simulink model "controlevento"  (Simulink 7.5)
settings: Solver=ode45  StartTime=0.0  StopTime=10000  RelTol=1e-3
values from neighbouring files (symbols this model uses):
  DL = tan(gamma0)*cos(sigma0)    [estressemain.m]    (also in main1.m)
  g = 9.81    [estressemain.m]    (also in main1.m)
  h0 = 5000    [estressemain.m]    (also in main1.m)
  href = 800    [estressemain.m]    (also in main1.m = 1000)
  meanw1 = 7    [estressemain.m]    (also in main1.m)
  meanw2 = 6    [estressemain.m]    (also in main1.m)
  meanw3 = 5    [estressemain.m]    (also in main1.m)
  meanw4 = 4    [estressemain.m]    (also in main1.m)
  meanw5 = 3    [estressemain.m]    (also in main1.m)
  psi0 = 360*(pi/180)    (= 6.28318530718)    [estressemain.m]    (also in main1.m)
  raioref = 400    [estressemain.m]    (also in main1.m)
  rhoH = 1.112    [estressemain.m]    (also in main1.m)
  rhoHo = 1.225    [estressemain.m]    (also in main1.m)
  Vo = 9    [estressemain.m]    (also in main1.m)
  wn = 1    [estressemain.m]    (also in main1.m = 150)
  x0 = 1000+i*rand    [estressemain.m]    (also in main1.m = 1000)
  xf = 0    [estressemain.m]    (also in main1.m = 500)
  y0 = 1000+i*rand    [estressemain.m]    (also in main1.m = 1000)
  yf = 0    [estressemain.m]    (also in main1.m)
  zm = 0.7    [estressemain.m]    (also in main1.m)
undefined symbols (not defined in the file or in its folder): fdesignblkfcn, gcbh
libraries: simulink x176, commnoisgen2 x10, dspsigops x1
(part 1 of 2)
settings Model: Creator=simonebattistini  LastModifiedBy=Yago Honda
settings DebuggingCC: SolverPrmCheckMsg=none  FcnCallInpInsideContextMsg=Enable All
settings GRTTargetCC: CombineOutputUpdateFcns=on

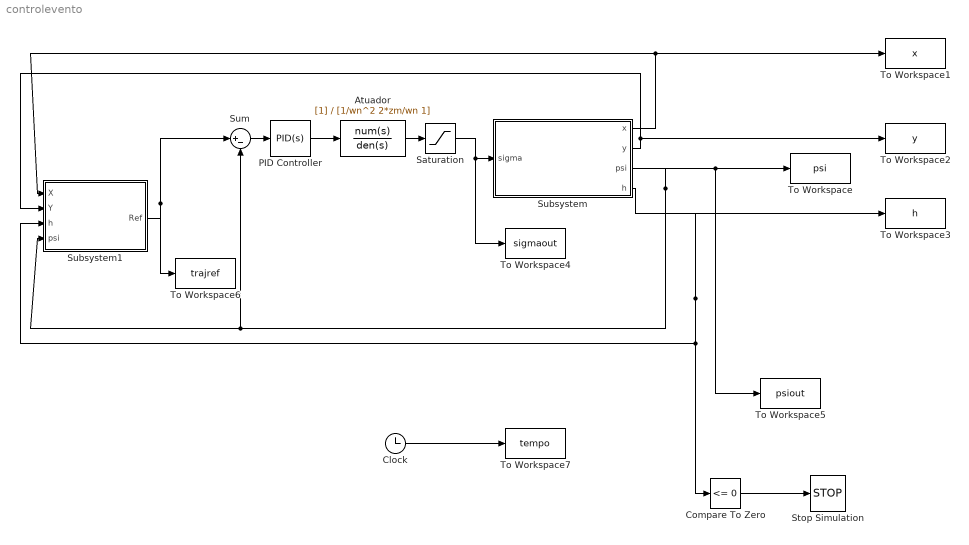
== system controlevento ==
  Atuador : TransferFcn  Denominator=[1/wn^2 2*zm/wn 1]  ContinuousStateAttributes='actuator'
  Clock : Clock
      settings: Decimation=10
  Compare To Zero : simulink/Logic and Bit Operations/Compare To Zero  SystemSampleTime=-1  relop=<=  LogicOutDataTypeMode=boolean
  PID Controller : simulink/Continuous/PID Controller  DialogController=pidpack.PIDConfig.pidDDGCreate  DialogControllerArgs=DataTag0  SystemSampleTime=-1  Controller=PID  TimeDomain=Continuous-time  SampleTime=1  IntegratorMethod=Forward Euler  FilterMethod=Forward Euler  Form=Parallel  P=-0.335721987396887  I=-0.000360400339747789  D=1.30119803967543  N=0.258009908684329  InitialConditionSource=internal  InitialConditionForIntegrator=0  InitialConditionForFilter=0  ExternalReset=none  LimitOutput=off  UpperSaturationLimit=inf  LowerSaturationLimit=-inf  LinearizeAsGain=off  AntiWindupMode=none  Kb=1  TrackingMode=off  Kt=1  PParamMin=[]  PParamMax=[]  IParamMin=[]  IParamMax=[]  DParamMin=[]  DParamMax=[]  NParamMin=[]  NParamMax=[]  KbParamMin=[]  KbParamMax=[]  KtParamMin=[]  KtParamMax=[]  POutMin=[]  POutMax=[]  IOutMin=[]  IOutMax=[]  DOutMin=[]  DOutMax=[]  NOutMin=[]  NOutMax=[]  KbOutMin=[]  KbOutMax=[]  KtOutMin=[]  KtOutMax=[]  IntegratorOutMin=[]  IntegratorOutMax=[]  FilterOutMin=[]  FilterOutMax=[]  SumOutMin=[]  SumOutMax=[]  SumI1OutMin=[]  SumI1OutMax=[]  SumI2OutMin=[]  SumI2OutMax=[]  SumI3OutMin=[]  SumI3OutMax=[]  SumDOutMin=[]  SumDOutMax=[]  SaturationOutMin=[]  SaturationOutMax=[]  IntegratorContinuousStateAttributes=''  IntegratorStateMustResolveToSignalObject=off  IntegratorRTWStateStorageClass=Auto  FilterContinuousStateAttributes=''  FilterStateMustResolveToSignalObject=off  FilterRTWStateStorageClass=Auto
  Saturation : Saturate  UpperLimit=20*pi/180  LowerLimit=-20*pi/180  OutDataType=fixdt(1, 16)  OutScaling=2^0
  Stop Simulation : Stop
  Subsystem : Subsystem
  Subsystem1 : Subsystem
  Sum : Sum  Inputs=|+-
  To Workspace : ToWorkspace  VariableName=psi  SampleTime=-1  SaveFormat=Array
  To Workspace1 : ToWorkspace  VariableName=x  SampleTime=-1  SaveFormat=Array
  To Workspace2 : ToWorkspace  VariableName=y  SampleTime=-1  SaveFormat=Array
  To Workspace3 : ToWorkspace  VariableName=h  SampleTime=-1  SaveFormat=Array
  To Workspace4 : ToWorkspace  VariableName=sigmaout  SampleTime=-1  SaveFormat=Array
  To Workspace5 : ToWorkspace  VariableName=psiout  SampleTime=-1  SaveFormat=Array
  To Workspace6 : ToWorkspace  VariableName=trajref  SampleTime=-1  SaveFormat=Array
  To Workspace7 : ToWorkspace  VariableName=tempo  SampleTime=-1  SaveFormat=Array
  wires:
  Sum/1 -> PID Controller/1
  Subsystem/3(psi) -> To Workspace5/1, To Workspace/1, Sum/2, Subsystem1/4(psi)
  Subsystem/1(x) -> Subsystem1/1(X), To Workspace1/1
  Subsystem/2(y) -> Subsystem1/2(Y), To Workspace2/1
  Subsystem/4(h) -> To Workspace3/1, Compare To Zero/1, Subsystem1/3(h)
  Subsystem1/1(Ref) -> Sum/1, To Workspace6/1
  Clock/1 -> To Workspace7/1
  Compare To Zero/1 -> Stop Simulation/1
  PID Controller/1 -> Atuador/1
  Saturation/1 -> Subsystem/1(sigma), To Workspace4/1
  Atuador/1 -> Saturation/1

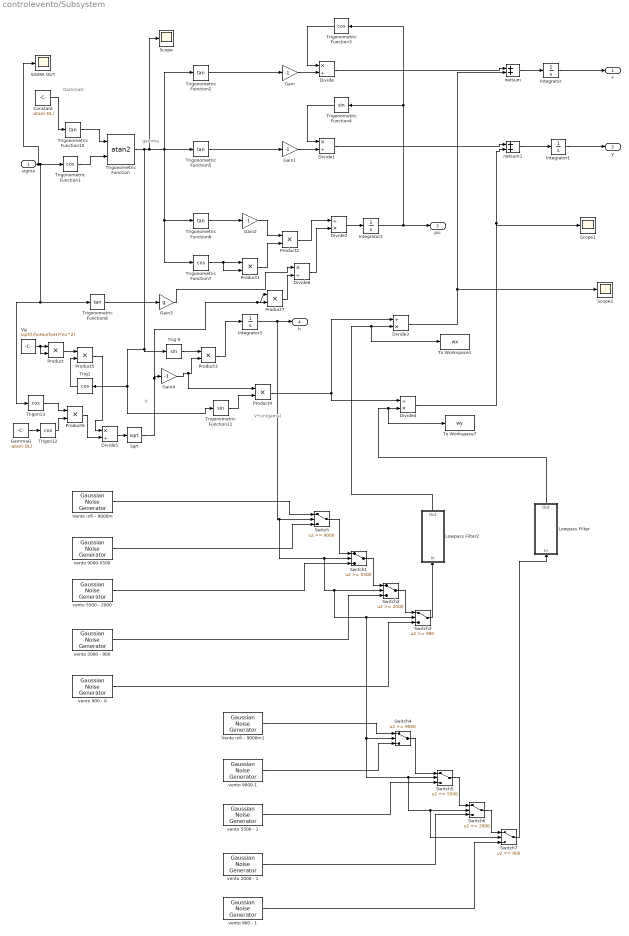
== system controlevento/Subsystem ==
  note: gamma
  note: V*sin(gama)
  note: GammaG
  note: V
  sigma : Inport
  Constant : Constant  Value=-atan(-DL)
  Divide{,1,5..6} (4 alike) : Product  Inputs=*/
  Divide2 : Product  Inputs=/*
  Divide3 : Product  Inputs=/*
  Divide4 : Product  Inputs=/*
  Gain{,1..2,4} (4 alike) : Gain  Gain=-1
  Gain3 : Gain  Gain=g
  GammaG : Constant  Value=-atan(-DL)
  Integrator : Integrator  InitialCondition=x0
  Integrator1 : Integrator  InitialCondition=y0
  Integrator2 : Integrator  InitialCondition=psi0
  Integrator3 : Integrator  InitialCondition=h0
  Lowpass Filter : Subsystem  DialogController=fdesignblkfcn  DialogControllerArgs=DataTag2  InitFcn=fdesignblkfcn(gcbh, {'InitFcn'});
      settings: CopyFcn=fdesignblkfcn(gcbh, {'CopyFcn'});
      mask Type: Lowpass Filter
      mask Description: Design a lowpass filter
      mask Help: helpview(mapfilelocation('dspblks'), 'dsplowpassfilter')
      mask Display: disp('Lowpass')
  Lowpass Filter2 : Subsystem  DialogController=fdesignblkfcn  DialogControllerArgs=DataTag5  InitFcn=fdesignblkfcn(gcbh, {'InitFcn'});
      settings: CopyFcn=fdesignblkfcn(gcbh, {'CopyFcn'});
      mask Type: Lowpass Filter
      mask Description: Design a lowpass filter
      mask Help: helpview(mapfilelocation('dspblks'), 'dsplowpassfilter')
      mask Display: disp('Lowpass')
  Product{,5..7} (4 alike) : Product  OutDataType=fixdt(1, 16)  OutScaling=2^0  RndMeth=Zero
  Product{1..4} (4 alike) : Product  RndMeth=Zero
  SIGMA OUT : Scope
      settings: SaveName=ScopeData4
  Scope : Scope
      settings: SaveName=ScopeData3
  Scope1 : Scope
      settings: SaveName=ScopeData7
  Scope2 : Scope
      settings: SaveName=ScopeData8
  Sqrt : Sqrt  SaturateOnIntegerOverflow=on
  Switch : Switch  Threshold=9000  OutDataType=fixdt(1, 16)  OutScaling=2^0
  Switch1 : Switch  Threshold=5500  OutDataType=fixdt(1, 16)  OutScaling=2^0
  Switch2 : Switch  Threshold=2000  OutDataType=fixdt(1, 16)  OutScaling=2^0
  Switch3 : Switch  Threshold=900  OutDataType=fixdt(1, 16)  OutScaling=2^0
  Switch4 : Switch  Threshold=9000  OutDataType=fixdt(1, 16)  OutScaling=2^0
  Switch5 : Switch  Threshold=5500  OutDataType=fixdt(1, 16)  OutScaling=2^0
  Switch6 : Switch  Threshold=2000  OutDataType=fixdt(1, 16)  OutScaling=2^0
  Switch7 : Switch  Threshold=900  OutDataType=fixdt(1, 16)  OutScaling=2^0
  To Workspace1 : ToWorkspace  VariableName=wx  SampleTime=-1  SaveFormat=Array
  To Workspace7 : ToWorkspace  VariableName=wy  SampleTime=-1  SaveFormat=Array
  Trig 9 : Trigonometry
  Trig1 : Trigonometry  Operator=cos
  Trigon12 : Trigonometry  Operator=cos
  Trigon13 : Trigonometry  Operator=cos
  Trigonometric Function : Trigonometry  Operator=atan2
  Trigonometric Function1 : Trigonometry  Operator=cos
  Trigonometric Function{2,5..6,8,10} (5 alike) : Trigonometry  Operator=tan
  Trigonometric Function11 : Trigonometry
  Trigonometric Function3 : Trigonometry  Operator=cos
  Trigonometric Function4 : Trigonometry
  Trigonometric Function7 : Trigonometry  Operator=cos
  Vento infi - 9000m : commnoisgen2/Gaussian Noise Generator  SystemSampleTime=-1  m=meanw1  d=varw1  s=seed1  Ts=1  frameBased=off  sampPerFrame=1  orient=off  outDataType=double
  Vento infi - 9000m1 : commnoisgen2/Gaussian Noise Generator  SystemSampleTime=-1  m=meanw1  d=varw1  s=seed1  Ts=2  frameBased=off  sampPerFrame=1  orient=off  outDataType=double
  Vg : Constant  Value=sqrt((rhoHo/rhoH)*Vo^2)
  netsum : Sum  Inputs=2  OutDataType=sfix(16)  OutScaling=2^0  SaturateOnIntegerOverflow=on  InputSameDT=on  OutDataTypeStr=Inherit: Same as first input
  netsum1 : Sum  Inputs=2  OutDataType=sfix(16)  OutScaling=2^0  SaturateOnIntegerOverflow=on  InputSameDT=on  OutDataTypeStr=Inherit: Same as first input
  vento 2000 - 1 : commnoisgen2/Gaussian Noise Generator  SystemSampleTime=-1  m=meanw4  d=varw4  s=seed4  Ts=1  frameBased=off  sampPerFrame=1  orient=off  outDataType=double
  vento 2000 - 900 : commnoisgen2/Gaussian Noise Generator  SystemSampleTime=-1  m=meanw4  d=varw4  s=seed4  Ts=1  frameBased=off  sampPerFrame=1  orient=off  outDataType=double
  vento 5500 - 1 : commnoisgen2/Gaussian Noise Generator  SystemSampleTime=-1  m=meanw3  d=varw3  s=seed3  Ts=1  frameBased=off  sampPerFrame=1  orient=off  outDataType=double
  vento 5500 - 2000 : commnoisgen2/Gaussian Noise Generator  SystemSampleTime=-1  m=meanw3  d=varw3  s=seed3  Ts=1  frameBased=off  sampPerFrame=1  orient=off  outDataType=double
  vento 900 - 0 : commnoisgen2/Gaussian Noise Generator  SystemSampleTime=-1  m=meanw5  d=varw5  s=seed5  Ts=1  frameBased=off  sampPerFrame=1  orient=off  outDataType=double
  vento 900 - 1 : commnoisgen2/Gaussian Noise Generator  SystemSampleTime=-1  m=meanw5  d=varw5  s=seed5  Ts=1  frameBased=off  sampPerFrame=1  orient=off  outDataType=double
  vento 9000-1 : commnoisgen2/Gaussian Noise Generator  SystemSampleTime=-1  m=meanw2  d=varw2  s=seed2  Ts=1  frameBased=off  sampPerFrame=1  orient=off  outDataType=double
  vento 9000-5500 : commnoisgen2/Gaussian Noise Generator  SystemSampleTime=-1  m=meanw2  d=varw2  s=seed2  Ts=1  frameBased=off  sampPerFrame=1  orient=off  outDataType=double
  x : Outport
  y : Outport  Port=2
  psi : Outport  Port=3
  h : Outport  Port=4
  wires:
  Integrator/1 -> x/1
  Integrator1/1 -> y/1
  Integrator2/1 -> Trigonometric Function3/1, Trigonometric Function4/1, psi/1
  sigma/1 -> Trigonometric Function1/1, Trigonometric Function8/1, Trigon13/1, SIGMA OUT/1
  Trigonometric Function1/1 -> Trigonometric Function/2
  Trigonometric Function/1 -> Trigonometric Function2/1, Trigonometric Function5/1, Trigonometric Function6/1, Trigonometric Function7/1, Scope/1, Trig 9/1, Trigonometric Function11/1, Trig1/1
  Trigonometric Function3/1 -> Divide/1
  Trigonometric Function2/1 -> Gain/1
  Gain/1 -> Divide/2
  Trigonometric Function5/1 -> Gain1/1
  Gain1/1 -> Divide1/2
  Trigonometric Function4/1 -> Divide1/1
  Trigonometric Function6/1 -> Gain2/1
  Divide2/1 -> Integrator2/1
  Trigonometric Function7/1 -> Product1/1, Product1/2
  Trigonometric Function8/1 -> Gain3/1
  Gain2/1 -> Product2/1
  Product1/1 -> Product2/2
  Product2/1 -> Divide2/1
  Trig 9/1 -> Product3/1
  Gain4/1 -> Product3/2, Product4/1
  Product3/1 -> Integrator3/1
  Integrator3/1 -> h/1, Switch/2, Switch1/2, Switch2/2, Switch3/2, Switch4/2, Switch5/2, Switch6/2, Switch7/2
  Constant/1 -> Trigonometric Function10/1
  Trigonometric Function10/1 -> Trigonometric Function/1
  Trigonometric Function11/1 -> Product4/2
  Product4/1 -> Divide3/1, Divide4/1
  netsum/1 -> Integrator/1
  netsum1/1 -> Integrator1/1
  Divide/1 -> netsum/1
  Divide1/1 -> netsum1/1
  Divide3/1 -> netsum/2, Scope2/1
  Divide4/1 -> netsum1/2, Scope1/1
  Vento infi - 9000m/1 -> Switch/1
  vento 9000-5500/1 -> Switch/3
  Switch/1 -> Switch1/1
  vento 5500 - 2000/1 -> Switch1/3
  vento 2000 - 900/1 -> Switch2/3
  Switch1/1 -> Switch2/1
  vento 900 - 0/1 -> Switch3/3
  Switch2/1 -> Switch3/1
  Vento infi - 9000m1/1 -> Switch4/1
  vento 9000-1/1 -> Switch4/3
  Switch4/1 -> Switch5/1
  vento 5500 - 1/1 -> Switch5/3
  vento 2000 - 1/1 -> Switch6/3
  Switch5/1 -> Switch6/1
  vento 900 - 1/1 -> Switch7/3
  Switch6/1 -> Switch7/1
  Switch3/1 -> Lowpass Filter2/1(In)
  Vg/1 -> Product/1, Product/2
  Product/1 -> Product5/1
  GammaG/1 -> Trigon12/1
  Trigon13/1 -> Product6/1
  Trigon12/1 -> Product6/2
  Trig1/1 -> Product5/2
  Product6/1 -> Divide5/2
  Product5/1 -> Divide5/1
  Divide5/1 -> Sqrt/1
  Sqrt/1 -> Gain4/1, Product7/1, Product7/2
  Gain3/1 -> Divide6/1
  Product7/1 -> Divide6/2
  Divide6/1 -> Divide2/2
  Switch7/1 -> Lowpass Filter/1(In)
  Lowpass Filter/1(Out) -> Divide4/2, To Workspace7/1
  Lowpass Filter2/1(Out) -> Divide3/2, To Workspace1/1

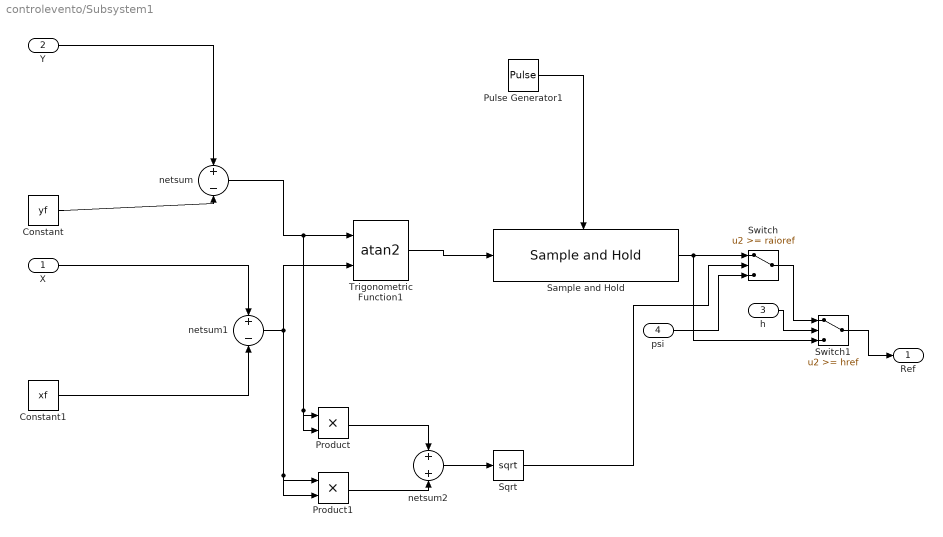
== system controlevento/Subsystem1 ==
  X : Inport  OutDataType=fixdt(1, 16)  OutScaling=2^0
  Y : Inport  Port=2  OutDataType=fixdt(1, 16)  OutScaling=2^0
  h : Inport  Port=3  OutDataType=fixdt(1, 16)  OutScaling=2^0
  psi : Inport  Port=4  OutDataType=fixdt(1, 16)  OutScaling=2^0
  Constant : Constant  Value=yf  OutDataType=fixdt(1, 16)  OutScaling=2^0
  Constant1 : Constant  Value=xf  OutDataType=fixdt(1, 16)  OutScaling=2^0
  Product : Product  OutDataType=fixdt(1, 16)  OutScaling=2^0  RndMeth=Zero
  Product1 : Product  OutDataType=fixdt(1, 16)  OutScaling=2^0  RndMeth=Zero
  Pulse Generator1 : DiscretePulseGenerator  PulseType=Time based  Amplitude=1  Period=3  PulseWidth=80  PhaseDelay=0  SampleTime=1
  Sample and Hold : dspsigops/Sample and Hold  SystemSampleTime=-1  trig=Rising edge  initCond=0  latchinput=on
  Sqrt : Sqrt  SaturateOnIntegerOverflow=on
  Switch : Switch  Threshold=raioref  OutDataType=fixdt(1, 16)  OutScaling=2^0
  Switch1 : Switch  Threshold=href  OutDataType=fixdt(1, 16)  OutScaling=2^0
  Trigonometric Function1 : Trigonometry  Operator=atan2
  netsum : Sum  Inputs=+|-  OutDataType=sfix(16)  OutScaling=2^0  SaturateOnIntegerOverflow=on  InputSameDT=on  OutDataTypeStr=Inherit: Same as first input
  netsum1 : Sum  Inputs=+|-  OutDataType=sfix(16)  OutScaling=2^0  SaturateOnIntegerOverflow=on  InputSameDT=on  OutDataTypeStr=Inherit: Same as first input
  netsum2 : Sum  Inputs=+|+  OutDataType=sfix(16)  OutScaling=2^0  SaturateOnIntegerOverflow=on  InputSameDT=on  OutDataTypeStr=Inherit: Same as first input
  Ref : Outport  OutDataType=fixdt(1, 16)  OutScaling=2^0
  wires:
  Constant/1 -> netsum/2
  Constant1/1 -> netsum1/2
  Y/1 -> netsum/1
  X/1 -> netsum1/1
  netsum/1 -> Trigonometric Function1/1, Product/1, Product/2
  netsum1/1 -> Trigonometric Function1/2, Product1/1, Product1/2
  Trigonometric Function1/1 -> Sample and Hold/1
  Pulse Generator1/1 -> Sample and Hold/Trigger
  Sample and Hold/1 -> Switch/1, Switch1/3
  psi/1 -> Switch/3
  Product1/1 -> netsum2/2
  Product/1 -> netsum2/1
  netsum2/1 -> Sqrt/1
  Sqrt/1 -> Switch/2
  h/1 -> Switch1/2
  Switch/1 -> Switch1/1
  Switch1/1 -> Ref/1

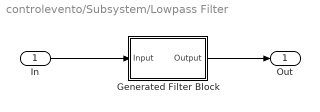
== system controlevento/Subsystem/Lowpass Filter ==
  In : Inport  OutDataType=sfix(16)  OutScaling=2^0
  Generated Filter Block : Subsystem  Tag=FilterWizardSubSystem
      settings: ErrorFcn=dspFilterRealizedInBasicElemsAlgLoopErrFcnCallback
  Out : Outport  OutDataType=sfix(16)  OutScaling=2^0
  wires:
  In/1 -> Generated Filter Block/1(Input)
  Generated Filter Block/1(Output) -> Out/1

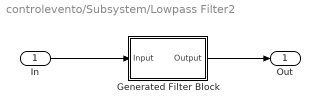
== system controlevento/Subsystem/Lowpass Filter2 ==
  In : Inport  OutDataType=sfix(16)  OutScaling=2^0
  Generated Filter Block : Subsystem  Tag=FilterWizardSubSystem
      settings: ErrorFcn=dspFilterRealizedInBasicElemsAlgLoopErrFcnCallback
  Out : Outport  OutDataType=sfix(16)  OutScaling=2^0
  wires:
  In/1 -> Generated Filter Block/1(Input)
  Generated Filter Block/1(Output) -> Out/1

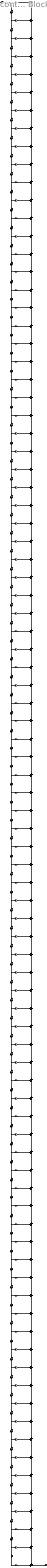
== system controlevento/Subsystem/Lowpass Filter/Generated Filter Block ==
  Input : Inport
  BodyDelay{2..88} (87 alike) : simulink/Discrete/Integer Delay  vinit=0  samptime=-1  NumDelays=1
  BodyLSum{2..88} (87 alike) : Sum  Inputs=++|  OutScaling=1  RndMeth=Nearest  SaturateOnIntegerOverflow=on  OutDataTypeStr=Inherit: Same as first input
  b(1) : Gain  Gain=0.00082164650590269158  ParameterDataTypeMode=Specify via dialog  ParameterDataType=float('double')  ParamDataTypeStr=float('double')  OutScaling=1  RndMeth=Nearest  SaturateOnIntegerOverflow=on  OutDataTypeStr=Inherit: Same as input
  b(10) : Gain  Gain=-0.0024182999746527817  ParameterDataTypeMode=Specify via dialog  ParameterDataType=float('double')  ParamDataTypeStr=float('double')  OutScaling=1  RndMeth=Nearest  SaturateOnIntegerOverflow=on  OutDataTypeStr=Inherit: Same as input
  b(11) : Gain  Gain=-0.0039635062129585018  ParameterDataTypeMode=Specify via dialog  ParameterDataType=float('double')  ParamDataTypeStr=float('double')  OutScaling=1  RndMeth=Nearest  SaturateOnIntegerOverflow=on  OutDataTypeStr=Inherit: Same as input
  b(12) : Gain  Gain=-0.0054910367027735324  ParameterDataTypeMode=Specify via dialog  ParameterDataType=float('double')  ParamDataTypeStr=float('double')  OutScaling=1  RndMeth=Nearest  SaturateOnIntegerOverflow=on  OutDataTypeStr=Inherit: Same as input
  b(13) : Gain  Gain=-0.0067921174004371976  ParameterDataTypeMode=Specify via dialog  ParameterDataType=float('double')  ParamDataTypeStr=float('double')  OutScaling=1  RndMeth=Nearest  SaturateOnIntegerOverflow=on  OutDataTypeStr=Inherit: Same as input
  b(14) : Gain  Gain=-0.0076451537219203317  ParameterDataTypeMode=Specify via dialog  ParameterDataType=float('double')  ParamDataTypeStr=float('double')  OutScaling=1  RndMeth=Nearest  SaturateOnIntegerOverflow=on  OutDataTypeStr=Inherit: Same as input
  b(15) : Gain  Gain=-0.0078449722479751478  ParameterDataTypeMode=Specify via dialog  ParameterDataType=float('double')  ParamDataTypeStr=float('double')  OutScaling=1  RndMeth=Nearest  SaturateOnIntegerOverflow=on  OutDataTypeStr=Inherit: Same as input
  b(16) : Gain  Gain=-0.0072402722086217083  ParameterDataTypeMode=Specify via dialog  ParameterDataType=float('double')  ParamDataTypeStr=float('double')  OutScaling=1  RndMeth=Nearest  SaturateOnIntegerOverflow=on  OutDataTypeStr=Inherit: Same as input
  b(17) : Gain  Gain=-0.0057663114777385654  ParameterDataTypeMode=Specify via dialog  ParameterDataType=float('double')  ParamDataTypeStr=float('double')  OutScaling=1  RndMeth=Nearest  SaturateOnIntegerOverflow=on  OutDataTypeStr=Inherit: Same as input
  b(18) : Gain  Gain=-0.0034705994320443937  ParameterDataTypeMode=Specify via dialog  ParameterDataType=float('double')  ParamDataTypeStr=float('double')  OutScaling=1  RndMeth=Nearest  SaturateOnIntegerOverflow=on  OutDataTypeStr=Inherit: Same as input
  b(19) : Gain  Gain=-0.00052529150396876515  ParameterDataTypeMode=Specify via dialog  ParameterDataType=float('double')  ParamDataTypeStr=float('double')  OutScaling=1  RndMeth=Nearest  SaturateOnIntegerOverflow=on  OutDataTypeStr=Inherit: Same as input
  b(2) : Gain  Gain=0.00086022764824789284  ParameterDataTypeMode=Specify via dialog  ParameterDataType=float('double')  ParamDataTypeStr=float('double')  OutScaling=1  RndMeth=Nearest  SaturateOnIntegerOverflow=on  OutDataTypeStr=Inherit: Same as input
  b(20) : Gain  Gain=0.0027734199688714718  ParameterDataTypeMode=Specify via dialog  ParameterDataType=float('double')  ParamDataTypeStr=float('double')  OutScaling=1  RndMeth=Nearest  SaturateOnIntegerOverflow=on  OutDataTypeStr=Inherit: Same as input
  b(21) : Gain  Gain=0.0060287364083220982  ParameterDataTypeMode=Specify via dialog  ParameterDataType=float('double')  ParamDataTypeStr=float('double')  OutScaling=1  RndMeth=Nearest  SaturateOnIntegerOverflow=on  OutDataTypeStr=Inherit: Same as input
  b(22) : Gain  Gain=0.0087841481976831393  ParameterDataTypeMode=Specify via dialog  ParameterDataType=float('double')  ParamDataTypeStr=float('double')  OutScaling=1  RndMeth=Nearest  SaturateOnIntegerOverflow=on  OutDataTypeStr=Inherit: Same as input
  b(23) : Gain  Gain=0.010578768801263436  ParameterDataTypeMode=Specify via dialog  ParameterDataType=float('double')  ParamDataTypeStr=float('double')  OutScaling=1  RndMeth=Nearest  SaturateOnIntegerOverflow=on  OutDataTypeStr=Inherit: Same as input
  b(24) : Gain  Gain=0.011013137679846739  ParameterDataTypeMode=Specify via dialog  ParameterDataType=float('double')  ParamDataTypeStr=float('double')  OutScaling=1  RndMeth=Nearest  SaturateOnIntegerOverflow=on  OutDataTypeStr=Inherit: Same as input
  b(25) : Gain  Gain=0.0098154176787387439  ParameterDataTypeMode=Specify via dialog  ParameterDataType=float('double')  ParamDataTypeStr=float('double')  OutScaling=1  RndMeth=Nearest  SaturateOnIntegerOverflow=on  OutDataTypeStr=Inherit: Same as input
  b(26) : Gain  Gain=0.0069012100728225619  ParameterDataTypeMode=Specify via dialog  ParameterDataType=float('double')  ParamDataTypeStr=float('double')  OutScaling=1  RndMeth=Nearest  SaturateOnIntegerOverflow=on  OutDataTypeStr=Inherit: Same as input
  b(27) : Gain  Gain=0.0024151501021086388  ParameterDataTypeMode=Specify via dialog  ParameterDataType=float('double')  ParamDataTypeStr=float('double')  OutScaling=1  RndMeth=Nearest  SaturateOnIntegerOverflow=on  OutDataTypeStr=Inherit: Same as input
  b(28) : Gain  Gain=-0.0032525081722248909  ParameterDataTypeMode=Specify via dialog  ParameterDataType=float('double')  ParamDataTypeStr=float('double')  OutScaling=1  RndMeth=Nearest  SaturateOnIntegerOverflow=on  OutDataTypeStr=Inherit: Same as input
  b(29) : Gain  Gain=-0.0094806769664186764  ParameterDataTypeMode=Specify via dialog  ParameterDataType=float('double')  ParamDataTypeStr=float('double')  OutScaling=1  RndMeth=Nearest  SaturateOnIntegerOverflow=on  OutDataTypeStr=Inherit: Same as input
  b(3) : Gain  Gain=0.0011651570184564182  ParameterDataTypeMode=Specify via dialog  ParameterDataType=float('double')  ParamDataTypeStr=float('double')  OutScaling=1  RndMeth=Nearest  SaturateOnIntegerOverflow=on  OutDataTypeStr=Inherit: Same as input
  b(30) : Gain  Gain=-0.0154628701847257  ParameterDataTypeMode=Specify via dialog  ParameterDataType=float('double')  ParamDataTypeStr=float('double')  OutScaling=1  RndMeth=Nearest  SaturateOnIntegerOverflow=on  OutDataTypeStr=Inherit: Same as input
  b(31) : Gain  Gain=-0.020282304307394423  ParameterDataTypeMode=Specify via dialog  ParameterDataType=float('double')  ParamDataTypeStr=float('double')  OutScaling=1  RndMeth=Nearest  SaturateOnIntegerOverflow=on  OutDataTypeStr=Inherit: Same as input
  b(32) : Gain  Gain=-0.023010638452223339  ParameterDataTypeMode=Specify via dialog  ParameterDataType=float('double')  ParamDataTypeStr=float('double')  OutScaling=1  RndMeth=Nearest  SaturateOnIntegerOverflow=on  OutDataTypeStr=Inherit: Same as input
  b(33) : Gain  Gain=-0.022817836498514321  ParameterDataTypeMode=Specify via dialog  ParameterDataType=float('double')  ParamDataTypeStr=float('double')  OutScaling=1  RndMeth=Nearest  SaturateOnIntegerOverflow=on  OutDataTypeStr=Inherit: Same as input
  b(34) : Gain  Gain=-0.01908164902026253  ParameterDataTypeMode=Specify via dialog  ParameterDataType=float('double')  ParamDataTypeStr=float('double')  OutScaling=1  RndMeth=Nearest  SaturateOnIntegerOverflow=on  OutDataTypeStr=Inherit: Same as input
  b(35) : Gain  Gain=-0.011481809355229307  ParameterDataTypeMode=Specify via dialog  ParameterDataType=float('double')  ParamDataTypeStr=float('double')  OutScaling=1  RndMeth=Nearest  SaturateOnIntegerOverflow=on  OutDataTypeStr=Inherit: Same as input
  b(36) : Gain  Gain=-6.6916305326006863e-005  ParameterDataTypeMode=Specify via dialog  ParameterDataType=float('double')  ParamDataTypeStr=float('double')  OutScaling=1  RndMeth=Nearest  SaturateOnIntegerOverflow=on  OutDataTypeStr=Inherit: Same as input
  b(37) : Gain  Gain=0.014717240662533493  ParameterDataTypeMode=Specify via dialog  ParameterDataType=float('double')  ParamDataTypeStr=float('double')  OutScaling=1  RndMeth=Nearest  SaturateOnIntegerOverflow=on  OutDataTypeStr=Inherit: Same as input
  b(38) : Gain  Gain=0.032042911444212341  ParameterDataTypeMode=Specify via dialog  ParameterDataType=float('double')  ParamDataTypeStr=float('double')  OutScaling=1  RndMeth=Nearest  SaturateOnIntegerOverflow=on  OutDataTypeStr=Inherit: Same as input
  b(39) : Gain  Gain=0.050760407285599524  ParameterDataTypeMode=Specify via dialog  ParameterDataType=float('double')  ParamDataTypeStr=float('double')  OutScaling=1  RndMeth=Nearest  SaturateOnIntegerOverflow=on  OutDataTypeStr=Inherit: Same as input
  b(4) : Gain  Gain=0.0013980355497406091  ParameterDataTypeMode=Specify via dialog  ParameterDataType=float('double')  ParamDataTypeStr=float('double')  OutScaling=1  RndMeth=Nearest  SaturateOnIntegerOverflow=on  OutDataTypeStr=Inherit: Same as input
  b(40) : Gain  Gain=0.069498244246696067  ParameterDataTypeMode=Specify via dialog  ParameterDataType=float('double')  ParamDataTypeStr=float('double')  OutScaling=1  RndMeth=Nearest  SaturateOnIntegerOverflow=on  OutDataTypeStr=Inherit: Same as input
  b(41) : Gain  Gain=0.086792739530761678  ParameterDataTypeMode=Specify via dialog  ParameterDataType=float('double')  ParamDataTypeStr=float('double')  OutScaling=1  RndMeth=Nearest  SaturateOnIntegerOverflow=on  OutDataTypeStr=Inherit: Same as input
  b(42) : Gain  Gain=0.10123382562240359  ParameterDataTypeMode=Specify via dialog  ParameterDataType=float('double')  ParamDataTypeStr=float('double')  OutScaling=1  RndMeth=Nearest  SaturateOnIntegerOverflow=on  OutDataTypeStr=Inherit: Same as input
  b(43) : Gain  Gain=0.11160927683175614  ParameterDataTypeMode=Specify via dialog  ParameterDataType=float('double')  ParamDataTypeStr=float('double')  OutScaling=1  RndMeth=Nearest  SaturateOnIntegerOverflow=on  OutDataTypeStr=Inherit: Same as input
  b(44) : Gain  Gain=0.11703150937672428  ParameterDataTypeMode=Specify via dialog  ParameterDataType=float('double')  ParamDataTypeStr=float('double')  OutScaling=1  RndMeth=Nearest  SaturateOnIntegerOverflow=on  OutDataTypeStr=Inherit: Same as input
  b(45) : Gain  Gain=0.11703150937672428  ParameterDataTypeMode=Specify via dialog  ParameterDataType=float('double')  ParamDataTypeStr=float('double')  OutScaling=1  RndMeth=Nearest  SaturateOnIntegerOverflow=on  OutDataTypeStr=Inherit: Same as input
  b(46) : Gain  Gain=0.11160927683175614  ParameterDataTypeMode=Specify via dialog  ParameterDataType=float('double')  ParamDataTypeStr=float('double')  OutScaling=1  RndMeth=Nearest  SaturateOnIntegerOverflow=on  OutDataTypeStr=Inherit: Same as input
  b(47) : Gain  Gain=0.10123382562240359  ParameterDataTypeMode=Specify via dialog  ParameterDataType=float('double')  ParamDataTypeStr=float('double')  OutScaling=1  RndMeth=Nearest  SaturateOnIntegerOverflow=on  OutDataTypeStr=Inherit: Same as input
  b(48) : Gain  Gain=0.086792739530761678  ParameterDataTypeMode=Specify via dialog  ParameterDataType=float('double')  ParamDataTypeStr=float('double')  OutScaling=1  RndMeth=Nearest  SaturateOnIntegerOverflow=on  OutDataTypeStr=Inherit: Same as input
  b(49) : Gain  Gain=0.069498244246696067  ParameterDataTypeMode=Specify via dialog  ParameterDataType=float('double')  ParamDataTypeStr=float('double')  OutScaling=1  RndMeth=Nearest  SaturateOnIntegerOverflow=on  OutDataTypeStr=Inherit: Same as input
  b(5) : Gain  Gain=0.0014794049503741346  ParameterDataTypeMode=Specify via dialog  ParameterDataType=float('double')  ParamDataTypeStr=float('double')  OutScaling=1  RndMeth=Nearest  SaturateOnIntegerOverflow=on  OutDataTypeStr=Inherit: Same as input
  b(50) : Gain  Gain=0.050760407285599524  ParameterDataTypeMode=Specify via dialog  ParameterDataType=float('double')  ParamDataTypeStr=float('double')  OutScaling=1  RndMeth=Nearest  SaturateOnIntegerOverflow=on  OutDataTypeStr=Inherit: Same as input
  b(51) : Gain  Gain=0.032042911444212341  ParameterDataTypeMode=Specify via dialog  ParameterDataType=float('double')  ParamDataTypeStr=float('double')  OutScaling=1  RndMeth=Nearest  SaturateOnIntegerOverflow=on  OutDataTypeStr=Inherit: Same as input
  b(52) : Gain  Gain=0.014717240662533493  ParameterDataTypeMode=Specify via dialog  ParameterDataType=float('double')  ParamDataTypeStr=float('double')  OutScaling=1  RndMeth=Nearest  SaturateOnIntegerOverflow=on  OutDataTypeStr=Inherit: Same as input
  b(53) : Gain  Gain=-6.6916305326006863e-005  ParameterDataTypeMode=Specify via dialog  ParameterDataType=float('double')  ParamDataTypeStr=float('double')  OutScaling=1  RndMeth=Nearest  SaturateOnIntegerOverflow=on  OutDataTypeStr=Inherit: Same as input
  b(54) : Gain  Gain=-0.011481809355229307  ParameterDataTypeMode=Specify via dialog  ParameterDataType=float('double')  ParamDataTypeStr=float('double')  OutScaling=1  RndMeth=Nearest  SaturateOnIntegerOverflow=on  OutDataTypeStr=Inherit: Same as input
  b(55) : Gain  Gain=-0.01908164902026253  ParameterDataTypeMode=Specify via dialog  ParameterDataType=float('double')  ParamDataTypeStr=float('double')  OutScaling=1  RndMeth=Nearest  SaturateOnIntegerOverflow=on  OutDataTypeStr=Inherit: Same as input
  b(56) : Gain  Gain=-0.022817836498514321  ParameterDataTypeMode=Specify via dialog  ParameterDataType=float('double')  ParamDataTypeStr=float('double')  OutScaling=1  RndMeth=Nearest  SaturateOnIntegerOverflow=on  OutDataTypeStr=Inherit: Same as input
  b(57) : Gain  Gain=-0.023010638452223339  ParameterDataTypeMode=Specify via dialog  ParameterDataType=float('double')  ParamDataTypeStr=float('double')  OutScaling=1  RndMeth=Nearest  SaturateOnIntegerOverflow=on  OutDataTypeStr=Inherit: Same as input
  b(58) : Gain  Gain=-0.020282304307394423  ParameterDataTypeMode=Specify via dialog  ParameterDataType=float('double')  ParamDataTypeStr=float('double')  OutScaling=1  RndMeth=Nearest  SaturateOnIntegerOverflow=on  OutDataTypeStr=Inherit: Same as input
  b(59) : Gain  Gain=-0.0154628701847257  ParameterDataTypeMode=Specify via dialog  ParameterDataType=float('double')  ParamDataTypeStr=float('double')  OutScaling=1  RndMeth=Nearest  SaturateOnIntegerOverflow=on  OutDataTypeStr=Inherit: Same as input
  b(6) : Gain  Gain=0.0013287887770783982  ParameterDataTypeMode=Specify via dialog  ParameterDataType=float('double')  ParamDataTypeStr=float('double')  OutScaling=1  RndMeth=Nearest  SaturateOnIntegerOverflow=on  OutDataTypeStr=Inherit: Same as input
  b(60) : Gain  Gain=-0.0094806769664186764  ParameterDataTypeMode=Specify via dialog  ParameterDataType=float('double')  ParamDataTypeStr=float('double')  OutScaling=1  RndMeth=Nearest  SaturateOnIntegerOverflow=on  OutDataTypeStr=Inherit: Same as input
  b(61) : Gain  Gain=-0.0032525081722248909  ParameterDataTypeMode=Specify via dialog  ParameterDataType=float('double')  ParamDataTypeStr=float('double')  OutScaling=1  RndMeth=Nearest  SaturateOnIntegerOverflow=on  OutDataTypeStr=Inherit: Same as input
  b(62) : Gain  Gain=0.0024151501021086388  ParameterDataTypeMode=Specify via dialog  ParameterDataType=float('double')  ParamDataTypeStr=float('double')  OutScaling=1  RndMeth=Nearest  SaturateOnIntegerOverflow=on  OutDataTypeStr=Inherit: Same as input
  b(63) : Gain  Gain=0.0069012100728225619  ParameterDataTypeMode=Specify via dialog  ParameterDataType=float('double')  ParamDataTypeStr=float('double')  OutScaling=1  RndMeth=Nearest  SaturateOnIntegerOverflow=on  OutDataTypeStr=Inherit: Same as input
  b(64) : Gain  Gain=0.0098154176787387439  ParameterDataTypeMode=Specify via dialog  ParameterDataType=float('double')  ParamDataTypeStr=float('double')  OutScaling=1  RndMeth=Nearest  SaturateOnIntegerOverflow=on  OutDataTypeStr=Inherit: Same as input
  b(65) : Gain  Gain=0.011013137679846739  ParameterDataTypeMode=Specify via dialog  ParameterDataType=float('double')  ParamDataTypeStr=float('double')  OutScaling=1  RndMeth=Nearest  SaturateOnIntegerOverflow=on  OutDataTypeStr=Inherit: Same as input
  b(66) : Gain  Gain=0.010578768801263436  ParameterDataTypeMode=Specify via dialog  ParameterDataType=float('double')  ParamDataTypeStr=float('double')  OutScaling=1  RndMeth=Nearest  SaturateOnIntegerOverflow=on  OutDataTypeStr=Inherit: Same as input
  b(67) : Gain  Gain=0.0087841481976831393  ParameterDataTypeMode=Specify via dialog  ParameterDataType=float('double')  ParamDataTypeStr=float('double')  OutScaling=1  RndMeth=Nearest  SaturateOnIntegerOverflow=on  OutDataTypeStr=Inherit: Same as input
  b(68) : Gain  Gain=0.0060287364083220982  ParameterDataTypeMode=Specify via dialog  ParameterDataType=float('double')  ParamDataTypeStr=float('double')  OutScaling=1  RndMeth=Nearest  SaturateOnIntegerOverflow=on  OutDataTypeStr=Inherit: Same as input
  b(69) : Gain  Gain=0.0027734199688714718  ParameterDataTypeMode=Specify via dialog  ParameterDataType=float('double')  ParamDataTypeStr=float('double')  OutScaling=1  RndMeth=Nearest  SaturateOnIntegerOverflow=on  OutDataTypeStr=Inherit: Same as input
  b(7) : Gain  Gain=0.00087870245058678347  ParameterDataTypeMode=Specify via dialog  ParameterDataType=float('double')  ParamDataTypeStr=float('double')  OutScaling=1  RndMeth=Nearest  SaturateOnIntegerOverflow=on  OutDataTypeStr=Inherit: Same as input
  b(70) : Gain  Gain=-0.00052529150396876515  ParameterDataTypeMode=Specify via dialog  ParameterDataType=float('double')  ParamDataTypeStr=float('double')  OutScaling=1  RndMeth=Nearest  SaturateOnIntegerOverflow=on  OutDataTypeStr=Inherit: Same as input
  b(71) : Gain  Gain=-0.0034705994320443937  ParameterDataTypeMode=Specify via dialog  ParameterDataType=float('double')  ParamDataTypeStr=float('double')  OutScaling=1  RndMeth=Nearest  SaturateOnIntegerOverflow=on  OutDataTypeStr=Inherit: Same as input
  b(72) : Gain  Gain=-0.0057663114777385654  ParameterDataTypeMode=Specify via dialog  ParameterDataType=float('double')  ParamDataTypeStr=float('double')  OutScaling=1  RndMeth=Nearest  SaturateOnIntegerOverflow=on  OutDataTypeStr=Inherit: Same as input
  b(73) : Gain  Gain=-0.0072402722086217083  ParameterDataTypeMode=Specify via dialog  ParameterDataType=float('double')  ParamDataTypeStr=float('double')  OutScaling=1  RndMeth=Nearest  SaturateOnIntegerOverflow=on  OutDataTypeStr=Inherit: Same as input
  b(74) : Gain  Gain=-0.0078449722479751478  ParameterDataTypeMode=Specify via dialog  ParameterDataType=float('double')  ParamDataTypeStr=float('double')  OutScaling=1  RndMeth=Nearest  SaturateOnIntegerOverflow=on  OutDataTypeStr=Inherit: Same as input
  b(75) : Gain  Gain=-0.0076451537219203317  ParameterDataTypeMode=Specify via dialog  ParameterDataType=float('double')  ParamDataTypeStr=float('double')  OutScaling=1  RndMeth=Nearest  SaturateOnIntegerOverflow=on  OutDataTypeStr=Inherit: Same as input
  b(76) : Gain  Gain=-0.0067921174004371976  ParameterDataTypeMode=Specify via dialog  ParameterDataType=float('double')  ParamDataTypeStr=float('double')  OutScaling=1  RndMeth=Nearest  SaturateOnIntegerOverflow=on  OutDataTypeStr=Inherit: Same as input
  b(77) : Gain  Gain=-0.0054910367027735324  ParameterDataTypeMode=Specify via dialog  ParameterDataType=float('double')  ParamDataTypeStr=float('double')  OutScaling=1  RndMeth=Nearest  SaturateOnIntegerOverflow=on  OutDataTypeStr=Inherit: Same as input
  b(78) : Gain  Gain=-0.0039635062129585018  ParameterDataTypeMode=Specify via dialog  ParameterDataType=float('double')  ParamDataTypeStr=float('double')  OutScaling=1  RndMeth=Nearest  SaturateOnIntegerOverflow=on  OutDataTypeStr=Inherit: Same as input
  b(79) : Gain  Gain=-0.0024182999746527817  ParameterDataTypeMode=Specify via dialog  ParameterDataType=float('double')  ParamDataTypeStr=float('double')  OutScaling=1  RndMeth=Nearest  SaturateOnIntegerOverflow=on  OutDataTypeStr=Inherit: Same as input
  b(8) : Gain  Gain=9.1668996700331904e-005  ParameterDataTypeMode=Specify via dialog  ParameterDataType=float('double')  ParamDataTypeStr=float('double')  OutScaling=1  RndMeth=Nearest  SaturateOnIntegerOverflow=on  OutDataTypeStr=Inherit: Same as input
  b(80) : Gain  Gain=-0.0010279120499869126  ParameterDataTypeMode=Specify via dialog  ParameterDataType=float('double')  ParamDataTypeStr=float('double')  OutScaling=1  RndMeth=Nearest  SaturateOnIntegerOverflow=on  OutDataTypeStr=Inherit: Same as input
  b(81) : Gain  Gain=9.1668996700331904e-005  ParameterDataTypeMode=Specify via dialog  ParameterDataType=float('double')  ParamDataTypeStr=float('double')  OutScaling=1  RndMeth=Nearest  SaturateOnIntegerOverflow=on  OutDataTypeStr=Inherit: Same as input
  b(82) : Gain  Gain=0.00087870245058678347  ParameterDataTypeMode=Specify via dialog  ParameterDataType=float('double')  ParamDataTypeStr=float('double')  OutScaling=1  RndMeth=Nearest  SaturateOnIntegerOverflow=on  OutDataTypeStr=Inherit: Same as input
  b(83) : Gain  Gain=0.0013287887770783982  ParameterDataTypeMode=Specify via dialog  ParameterDataType=float('double')  ParamDataTypeStr=float('double')  OutScaling=1  RndMeth=Nearest  SaturateOnIntegerOverflow=on  OutDataTypeStr=Inherit: Same as input
  b(84) : Gain  Gain=0.0014794049503741346  ParameterDataTypeMode=Specify via dialog  ParameterDataType=float('double')  ParamDataTypeStr=float('double')  OutScaling=1  RndMeth=Nearest  SaturateOnIntegerOverflow=on  OutDataTypeStr=Inherit: Same as input
  b(85) : Gain  Gain=0.0013980355497406091  ParameterDataTypeMode=Specify via dialog  ParameterDataType=float('double')  ParamDataTypeStr=float('double')  OutScaling=1  RndMeth=Nearest  SaturateOnIntegerOverflow=on  OutDataTypeStr=Inherit: Same as input
  b(86) : Gain  Gain=0.0011651570184564182  ParameterDataTypeMode=Specify via dialog  ParameterDataType=float('double')  ParamDataTypeStr=float('double')  OutScaling=1  RndMeth=Nearest  SaturateOnIntegerOverflow=on  OutDataTypeStr=Inherit: Same as input
  b(87) : Gain  Gain=0.00086022764824789284  ParameterDataTypeMode=Specify via dialog  ParameterDataType=float('double')  ParamDataTypeStr=float('double')  OutScaling=1  RndMeth=Nearest  SaturateOnIntegerOverflow=on  OutDataTypeStr=Inherit: Same as input
  b(88) : Gain  Gain=0.00082164650590269158  ParameterDataTypeMode=Specify via dialog  ParameterDataType=float('double')  ParamDataTypeStr=float('double')  OutScaling=1  RndMeth=Nearest  SaturateOnIntegerOverflow=on  OutDataTypeStr=Inherit: Same as input
  b(9) : Gain  Gain=-0.0010279120499869126  ParameterDataTypeMode=Specify via dialog  ParameterDataType=float('double')  ParamDataTypeStr=float('double')  OutScaling=1  RndMeth=Nearest  SaturateOnIntegerOverflow=on  OutDataTypeStr=Inherit: Same as input
  Output : Outport
  wires:
  Input/1 -> b(1)/1, BodyDelay2/1
  b(1)/1 -> BodyLSum2/2
  BodyDelay2/1 -> b(2)/1, BodyDelay3/1
  b(2)/1 -> BodyLSum2/1
  BodyLSum2/1 -> BodyLSum3/2
  BodyDelay3/1 -> b(3)/1, BodyDelay4/1
  b(3)/1 -> BodyLSum3/1
  BodyLSum3/1 -> BodyLSum4/2
  BodyDelay4/1 -> b(4)/1, BodyDelay5/1
  b(4)/1 -> BodyLSum4/1
  BodyLSum4/1 -> BodyLSum5/2
  BodyDelay5/1 -> b(5)/1, BodyDelay6/1
  b(5)/1 -> BodyLSum5/1
  BodyLSum5/1 -> BodyLSum6/2
  BodyDelay6/1 -> b(6)/1, BodyDelay7/1
  b(6)/1 -> BodyLSum6/1
  BodyLSum6/1 -> BodyLSum7/2
  BodyDelay7/1 -> b(7)/1, BodyDelay8/1
  b(7)/1 -> BodyLSum7/1
  BodyLSum7/1 -> BodyLSum8/2
  BodyDelay8/1 -> b(8)/1, BodyDelay9/1
  b(8)/1 -> BodyLSum8/1
  BodyLSum8/1 -> BodyLSum9/2
  BodyDelay9/1 -> b(9)/1, BodyDelay10/1
  b(9)/1 -> BodyLSum9/1
  BodyLSum9/1 -> BodyLSum10/2
  BodyDelay10/1 -> b(10)/1, BodyDelay11/1
  b(10)/1 -> BodyLSum10/1
  BodyLSum10/1 -> BodyLSum11/2
  BodyDelay11/1 -> b(11)/1, BodyDelay12/1
  b(11)/1 -> BodyLSum11/1
  BodyLSum11/1 -> BodyLSum12/2
  BodyDelay12/1 -> b(12)/1, BodyDelay13/1
  b(12)/1 -> BodyLSum12/1
  BodyLSum12/1 -> BodyLSum13/2
  BodyDelay13/1 -> b(13)/1, BodyDelay14/1
  b(13)/1 -> BodyLSum13/1
  BodyLSum13/1 -> BodyLSum14/2
  BodyDelay14/1 -> b(14)/1, BodyDelay15/1
  b(14)/1 -> BodyLSum14/1
  BodyLSum14/1 -> BodyLSum15/2
  BodyDelay15/1 -> b(15)/1, BodyDelay16/1
  b(15)/1 -> BodyLSum15/1
  BodyLSum15/1 -> BodyLSum16/2
  BodyDelay16/1 -> b(16)/1, BodyDelay17/1
  b(16)/1 -> BodyLSum16/1
  BodyLSum16/1 -> BodyLSum17/2
  BodyDelay17/1 -> b(17)/1, BodyDelay18/1
  b(17)/1 -> BodyLSum17/1
  BodyLSum17/1 -> BodyLSum18/2
  BodyDelay18/1 -> b(18)/1, BodyDelay19/1
  b(18)/1 -> BodyLSum18/1
  BodyLSum18/1 -> BodyLSum19/2
  BodyDelay19/1 -> b(19)/1, BodyDelay20/1
  b(19)/1 -> BodyLSum19/1
  BodyLSum19/1 -> BodyLSum20/2
  BodyDelay20/1 -> b(20)/1, BodyDelay21/1
  b(20)/1 -> BodyLSum20/1
  BodyLSum20/1 -> BodyLSum21/2
  BodyDelay21/1 -> b(21)/1, BodyDelay22/1
  b(21)/1 -> BodyLSum21/1
  BodyLSum21/1 -> BodyLSum22/2
  BodyDelay22/1 -> b(22)/1, BodyDelay23/1
  b(22)/1 -> BodyLSum22/1
  BodyLSum22/1 -> BodyLSum23/2
  BodyDelay23/1 -> b(23)/1, BodyDelay24/1
  b(23)/1 -> BodyLSum23/1
  BodyLSum23/1 -> BodyLSum24/2
  BodyDelay24/1 -> b(24)/1, BodyDelay25/1
  b(24)/1 -> BodyLSum24/1
  BodyLSum24/1 -> BodyLSum25/2
  BodyDelay25/1 -> b(25)/1, BodyDelay26/1
  b(25)/1 -> BodyLSum25/1
  BodyLSum25/1 -> BodyLSum26/2
  BodyDelay26/1 -> b(26)/1, BodyDelay27/1
  b(26)/1 -> BodyLSum26/1
  BodyLSum26/1 -> BodyLSum27/2
  BodyDelay27/1 -> b(27)/1, BodyDelay28/1
  b(27)/1 -> BodyLSum27/1
  BodyLSum27/1 -> BodyLSum28/2
  BodyDelay28/1 -> b(28)/1, BodyDelay29/1
  b(28)/1 -> BodyLSum28/1
  BodyLSum28/1 -> BodyLSum29/2
  BodyDelay29/1 -> b(29)/1, BodyDelay30/1
  b(29)/1 -> BodyLSum29/1
  BodyLSum29/1 -> BodyLSum30/2
  BodyDelay30/1 -> b(30)/1, BodyDelay31/1
  b(30)/1 -> BodyLSum30/1
  BodyLSum30/1 -> BodyLSum31/2
  BodyDelay31/1 -> b(31)/1, BodyDelay32/1
  b(31)/1 -> BodyLSum31/1
  BodyLSum31/1 -> BodyLSum32/2
  BodyDelay32/1 -> b(32)/1, BodyDelay33/1
  b(32)/1 -> BodyLSum32/1
  BodyLSum32/1 -> BodyLSum33/2
  BodyDelay33/1 -> b(33)/1, BodyDelay34/1
  b(33)/1 -> BodyLSum33/1
  BodyLSum33/1 -> BodyLSum34/2
  BodyDelay34/1 -> b(34)/1, BodyDelay35/1
  b(34)/1 -> BodyLSum34/1
  BodyLSum34/1 -> BodyLSum35/2
  BodyDelay35/1 -> b(35)/1, BodyDelay36/1
  b(35)/1 -> BodyLSum35/1
  BodyLSum35/1 -> BodyLSum36/2
  BodyDelay36/1 -> b(36)/1, BodyDelay37/1
  b(36)/1 -> BodyLSum36/1
  BodyLSum36/1 -> BodyLSum37/2
  BodyDelay37/1 -> b(37)/1, BodyDelay38/1
  b(37)/1 -> BodyLSum37/1
  BodyLSum37/1 -> BodyLSum38/2
  BodyDelay38/1 -> b(38)/1, BodyDelay39/1
  b(38)/1 -> BodyLSum38/1
  BodyLSum38/1 -> BodyLSum39/2
  BodyDelay39/1 -> b(39)/1, BodyDelay40/1
  b(39)/1 -> BodyLSum39/1
  BodyLSum39/1 -> BodyLSum40/2
  BodyDelay40/1 -> b(40)/1, BodyDelay41/1
  b(40)/1 -> BodyLSum40/1
  BodyLSum40/1 -> BodyLSum41/2
  BodyDelay41/1 -> b(41)/1, BodyDelay42/1
  b(41)/1 -> BodyLSum41/1
  BodyLSum41/1 -> BodyLSum42/2
  BodyDelay42/1 -> b(42)/1, BodyDelay43/1
  b(42)/1 -> BodyLSum42/1
  BodyLSum42/1 -> BodyLSum43/2
  BodyDelay43/1 -> b(43)/1, BodyDelay44/1
  b(43)/1 -> BodyLSum43/1
  BodyLSum43/1 -> BodyLSum44/2
  BodyDelay44/1 -> b(44)/1, BodyDelay45/1
  b(44)/1 -> BodyLSum44/1
  BodyLSum44/1 -> BodyLSum45/2
  BodyDelay45/1 -> b(45)/1, BodyDelay46/1
  b(45)/1 -> BodyLSum45/1
  BodyLSum45/1 -> BodyLSum46/2
  BodyDelay46/1 -> b(46)/1, BodyDelay47/1
  b(46)/1 -> BodyLSum46/1
  BodyLSum46/1 -> BodyLSum47/2
  BodyDelay47/1 -> b(47)/1, BodyDelay48/1
  b(47)/1 -> BodyLSum47/1
  BodyLSum47/1 -> BodyLSum48/2
  BodyDelay48/1 -> b(48)/1, BodyDelay49/1
  b(48)/1 -> BodyLSum48/1
  BodyLSum48/1 -> BodyLSum49/2
  BodyDelay49/1 -> b(49)/1, BodyDelay50/1
  b(49)/1 -> BodyLSum49/1
  BodyLSum49/1 -> BodyLSum50/2
  BodyDelay50/1 -> b(50)/1, BodyDelay51/1
  b(50)/1 -> BodyLSum50/1
  BodyLSum50/1 -> BodyLSum51/2
  BodyDelay51/1 -> b(51)/1, BodyDelay52/1
  b(51)/1 -> BodyLSum51/1
  BodyLSum51/1 -> BodyLSum52/2
  BodyDelay52/1 -> b(52)/1, BodyDelay53/1
  b(52)/1 -> BodyLSum52/1
  BodyLSum52/1 -> BodyLSum53/2
  BodyDelay53/1 -> b(53)/1, BodyDelay54/1
  b(53)/1 -> BodyLSum53/1
  BodyLSum53/1 -> BodyLSum54/2
  BodyDelay54/1 -> b(54)/1, BodyDelay55/1
  b(54)/1 -> BodyLSum54/1
  BodyLSum54/1 -> BodyLSum55/2
  BodyDelay55/1 -> b(55)/1, BodyDelay56/1
  b(55)/1 -> BodyLSum55/1
  BodyLSum55/1 -> BodyLSum56/2
  BodyDelay56/1 -> b(56)/1, BodyDelay57/1
  b(56)/1 -> BodyLSum56/1
  BodyLSum56/1 -> BodyLSum57/2
  BodyDelay57/1 -> b(57)/1, BodyDelay58/1
  b(57)/1 -> BodyLSum57/1
  BodyLSum57/1 -> BodyLSum58/2
  BodyDelay58/1 -> b(58)/1, BodyDelay59/1
  b(58)/1 -> BodyLSum58/1
  BodyLSum58/1 -> BodyLSum59/2
  BodyDelay59/1 -> b(59)/1, BodyDelay60/1
  b(59)/1 -> BodyLSum59/1
  BodyLSum59/1 -> BodyLSum60/2
  BodyDelay60/1 -> b(60)/1, BodyDelay61/1
  b(60)/1 -> BodyLSum60/1
  BodyLSum60/1 -> BodyLSum61/2
  BodyDelay61/1 -> b(61)/1, BodyDelay62/1
  b(61)/1 -> BodyLSum61/1
  BodyLSum61/1 -> BodyLSum62/2
  BodyDelay62/1 -> b(62)/1, BodyDelay63/1
  b(62)/1 -> BodyLSum62/1
  BodyLSum62/1 -> BodyLSum63/2
  BodyDelay63/1 -> b(63)/1, BodyDelay64/1
  b(63)/1 -> BodyLSum63/1
  BodyLSum63/1 -> BodyLSum64/2
  BodyDelay64/1 -> b(64)/1, BodyDelay65/1
  b(64)/1 -> BodyLSum64/1
  BodyLSum64/1 -> BodyLSum65/2
  BodyDelay65/1 -> b(65)/1, BodyDelay66/1
  b(65)/1 -> BodyLSum65/1
  BodyLSum65/1 -> BodyLSum66/2
  BodyDelay66/1 -> b(66)/1, BodyDelay67/1
  b(66)/1 -> BodyLSum66/1
  BodyLSum66/1 -> BodyLSum67/2
  BodyDelay67/1 -> b(67)/1, BodyDelay68/1
  b(67)/1 -> BodyLSum67/1
  BodyLSum67/1 -> BodyLSum68/2
  BodyDelay68/1 -> b(68)/1, BodyDelay69/1
  b(68)/1 -> BodyLSum68/1
  BodyLSum68/1 -> BodyLSum69/2
  BodyDelay69/1 -> b(69)/1, BodyDelay70/1
  b(69)/1 -> BodyLSum69/1
  BodyLSum69/1 -> BodyLSum70/2
  BodyDelay70/1 -> b(70)/1, BodyDelay71/1
  b(70)/1 -> BodyLSum70/1
  BodyLSum70/1 -> BodyLSum71/2
  BodyDelay71/1 -> b(71)/1, BodyDelay72/1
  b(71)/1 -> BodyLSum71/1
  BodyLSum71/1 -> BodyLSum72/2
  BodyDelay72/1 -> b(72)/1, BodyDelay73/1
  b(72)/1 -> BodyLSum72/1
  BodyLSum72/1 -> BodyLSum73/2
  BodyDelay73/1 -> b(73)/1, BodyDelay74/1
  b(73)/1 -> BodyLSum73/1
  BodyLSum73/1 -> BodyLSum74/2
  BodyDelay74/1 -> b(74)/1, BodyDelay75/1
  b(74)/1 -> BodyLSum74/1
  BodyLSum74/1 -> BodyLSum75/2
  BodyDelay75/1 -> b(75)/1, BodyDelay76/1
  b(75)/1 -> BodyLSum75/1
  BodyLSum75/1 -> BodyLSum76/2
  BodyDelay76/1 -> b(76)/1, BodyDelay77/1
  b(76)/1 -> BodyLSum76/1
  BodyLSum76/1 -> BodyLSum77/2
  BodyDelay77/1 -> b(77)/1, BodyDelay78/1
  b(77)/1 -> BodyLSum77/1
  BodyLSum77/1 -> BodyLSum78/2
  BodyDelay78/1 -> b(78)/1, BodyDelay79/1
  b(78)/1 -> BodyLSum78/1
  BodyLSum78/1 -> BodyLSum79/2
  BodyDelay79/1 -> b(79)/1, BodyDelay80/1
  b(79)/1 -> BodyLSum79/1
  BodyLSum79/1 -> BodyLSum80/2
  BodyDelay80/1 -> b(80)/1, BodyDelay81/1
  b(80)/1 -> BodyLSum80/1
  BodyLSum80/1 -> BodyLSum81/2
  BodyDelay81/1 -> b(81)/1, BodyDelay82/1
  b(81)/1 -> BodyLSum81/1
  BodyLSum81/1 -> BodyLSum82/2
  BodyDelay82/1 -> b(82)/1, BodyDelay83/1
  b(82)/1 -> BodyLSum82/1
  BodyLSum82/1 -> BodyLSum83/2
  BodyDelay83/1 -> b(83)/1, BodyDelay84/1
  b(83)/1 -> BodyLSum83/1
  BodyLSum83/1 -> BodyLSum84/2
  BodyDelay84/1 -> b(84)/1, BodyDelay85/1
  b(84)/1 -> BodyLSum84/1
  BodyLSum84/1 -> BodyLSum85/2
  BodyDelay85/1 -> b(85)/1, BodyDelay86/1
  b(85)/1 -> BodyLSum85/1
  BodyLSum85/1 -> BodyLSum86/2
  BodyDelay86/1 -> b(86)/1, BodyDelay87/1
  b(86)/1 -> BodyLSum86/1
  BodyLSum86/1 -> BodyLSum87/2
  BodyDelay87/1 -> b(87)/1, BodyDelay88/1
  b(87)/1 -> BodyLSum87/1
  BodyLSum87/1 -> BodyLSum88/1
  BodyDelay88/1 -> b(88)/1
  b(88)/1 -> BodyLSum88/2
  BodyLSum88/1 -> Output/1
